simulink model "pll__"  (Simulink 7.5)
settings: Solver=ode45  StartTime=0.0  StopTime=10.0  RelTol=1e-3
libraries: commsynccomp2 x2
CloseFcn:
  | rtwprivate ssgencode ModelCloseRequest pll__
settings Model: Creator=kostas777711  LastModifiedBy=kostas777711
settings RTWCC: ProcessScript=grt_make_rtw_hook

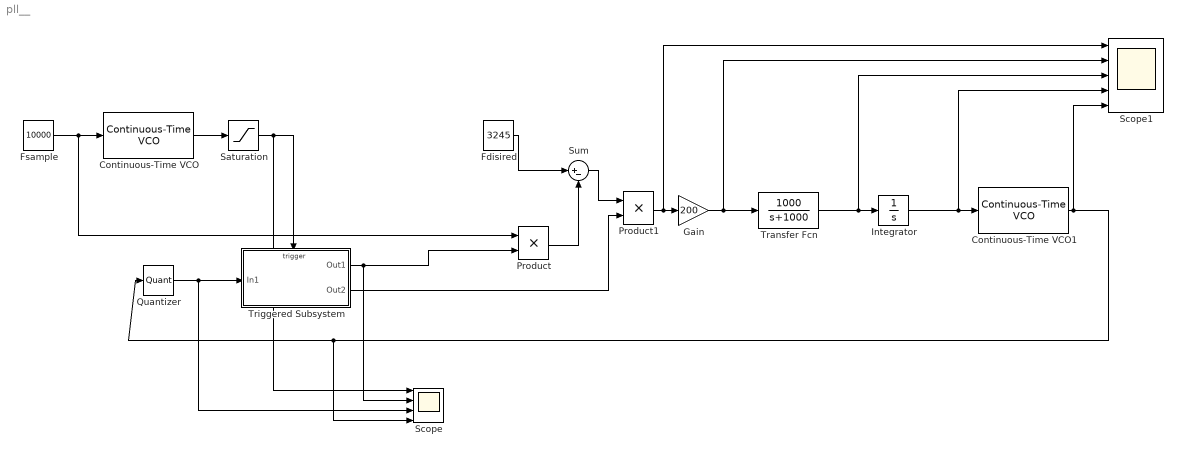
== system pll__ ==
  Continuous-Time VCO : commsynccomp2/Continuous-Time VCO  SystemSampleTime=-1  Ac=1  Fc=0  Kc=1  Ph=0
  Continuous-Time VCO1 : commsynccomp2/Continuous-Time VCO  SystemSampleTime=-1  Ac=1  Fc=0  Kc=1  Ph=0
  Fdisired : Constant  Value=3245  OutDataType=fixdt(1, 16)  OutScaling=2^0
  Fsample : Constant  Value=10000  OutDataType=fixdt(1, 16)  OutScaling=2^0
  Gain : Gain  Gain=200  ParameterDataType=fixdt(1, 16)  ParameterScaling=2^0  OutDataType=fixdt(1, 16)  OutScaling=2^0
  Integrator : Integrator
  Product : Product  OutDataType=fixdt(1, 16)  OutScaling=2^0  RndMeth=Zero
  Product1 : Product  OutDataType=fixdt(1, 16)  OutScaling=2^0  RndMeth=Zero
  Quantizer : Quantizer  QuantizationInterval=2/(2^8)
  Saturation : Saturate  UpperLimit=1  LowerLimit=-1  OutDataType=fixdt(1, 16)  OutScaling=2^0
  Scope : Scope  NumInputPorts=4
      settings: TimeRange=0.009174311926605505  YMin=-1~-1~-1~-1  YMax=1~1~1~1
  Scope1 : Scope  NumInputPorts=5
      settings: TimeRange=0.0007049700387733521  YMin=250~50000~380000~104050~-1  YMax=3250~650000~460000~104600~1
  Sum : Sum  Inputs=|+-  OutDataType=fixdt(1, 16)  OutScaling=2^0
  Transfer Fcn : TransferFcn  Numerator=[1000]  Denominator=[1 1000]
  Triggered Subsystem : Subsystem  TreatAsAtomicUnit=on
  wires:
  Fsample/1 -> Continuous-Time VCO/1, Product/1
  Continuous-Time VCO/1 -> Saturation/1
  Saturation/1 -> Triggered Subsystem/Trigger, Scope/1
  Quantizer/1 -> Triggered Subsystem/1(In1), Scope/3
  Triggered Subsystem/2(Out2) -> Product1/2
  Transfer Fcn/1 -> Integrator/1, Scope1/3
  Gain/1 -> Scope1/2, Transfer Fcn/1
  Fdisired/1 -> Sum/1
  Product/1 -> Sum/2
  Continuous-Time VCO1/1 -> Scope1/5, Quantizer/1, Scope/4
  Product1/1 -> Gain/1, Scope1/1
  Sum/1 -> Product1/1
  Triggered Subsystem/1(Out1) -> Product/2, Scope/2
  Integrator/1 -> Continuous-Time VCO1/1, Scope1/4

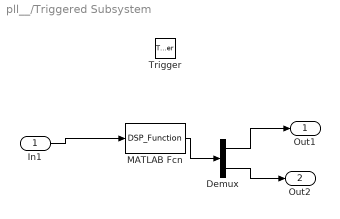
== system pll__/Triggered Subsystem ==
  In1 : Inport  OutDataType=fixdt(1, 16)  OutScaling=2^0
  Trigger : TriggerPort
  Demux : Demux  Outputs=2
  MATLAB Fcn : MATLABFcn  MATLABFcn=DSP_Function  OutputDimensions=2
  Out1 : Outport  OutDataType=fixdt(1, 16)  OutScaling=2^0
  Out2 : Outport  Port=2  OutDataType=fixdt(1, 16)  OutScaling=2^0
  wires:
  In1/1 -> MATLAB Fcn/1
  MATLAB Fcn/1 -> Demux/1
  Demux/1 -> Out1/1
  Demux/2 -> Out2/1
